simulink model "Compliance"  (R2020b)
settings: Solver=VariableStepAuto  StartTime=0.0  StopTime=3  RelTol=1e-3
values from neighbouring files (symbols this model uses):
  K = 10*diag([1 1 30 1 1 1])    [parameters.m]
  KD = diag([  150   180   160    19     0   8])    [parameters.m]
  KP = diag([1700  3000  1600  100  1  4])    [parameters.m]
libraries: vrlib x1
settings Model: Creator=Edoardo  LastModifiedBy=Edoardo

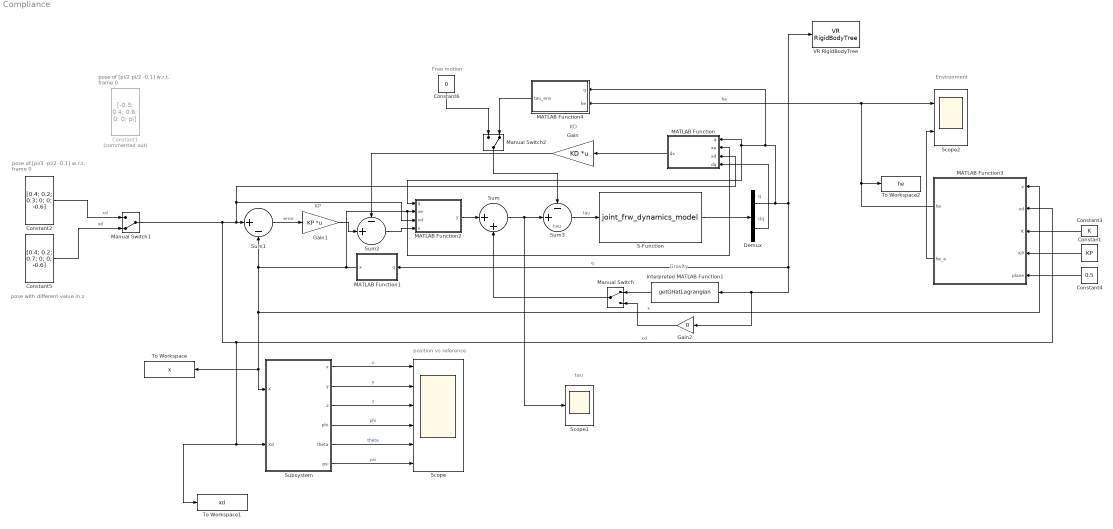
== system Compliance ==
  note: Free motion
  note: Environment
  note: tau
  note: Gravity
  note: tau
  note: KP
  note: KD
  note: dq
  note: q
  note: position vs reference
  note: pose of [pi/2 pi/2 -0.1]
      | w.r.t. frame 0
  note: pose of [pi/3 -pi/2 -0.1]
      | w.r.t. frame 0
  note: pose with different value in z
  Constant : Constant  Value=KP
  Constant1 : Constant  Commented=on  Value=[-0.3; 0.4; 0.6; 0; 0; pi]  VectorParams1D=off
  Constant2 : Constant  Value=[0.4; 0.2; 0.3; 0; 0; -0.6]  VectorParams1D=off
  Constant3 : Constant  Value=K
  Constant4 : Constant  Value=0.5
  Constant5 : Constant  Value=[0.4; 0.2; 0.7; 0; 0; -0.6]  VectorParams1D=off
  Constant6 : Constant  Value=0
  Demux : Demux  Outputs=2
  Gain : Gain  Gain=KD  Multiplication=Matrix(K*u) (u vector)
  Gain1 : Gain  Gain=KP  Multiplication=Matrix(K*u) (u vector)
  Gain2 : Gain  Gain=0
  Interpreted MATLAB Function1 : MATLABFcn  MATLABFcn=getGHatLagrangian
  MATLAB Function : MATLAB Function  TreatAsAtomicUnit=on
  MATLAB Function1 : MATLAB Function  TreatAsAtomicUnit=on
  MATLAB Function2 : MATLAB Function  TreatAsAtomicUnit=on
  MATLAB Function3 : MATLAB Function  TreatAsAtomicUnit=on
  MATLAB Function4 : MATLAB Function  TreatAsAtomicUnit=on
  Manual Switch : ManualSwitch
  Manual Switch1 : ManualSwitch  CurrentSetting=0
  Manual Switch2 : ManualSwitch  CurrentSetting=0
  S-Function : S-Function  FunctionName=joint_frw_dynamics_model  Parameters=myRobot  SFunctionDeploymentMode=off  EnableBusSupport=off
  Scope : Scope  NumInputPorts=6
  Scope1 : Scope
  Scope2 : Scope  NumInputPorts=2
  Subsystem : Subsystem
  Sum : Sum  Inputs=|++
  Sum1 : Sum  Inputs=|+-
  Sum2 : Sum  Inputs=-+|
  Sum3 : Sum  Inputs=-+|
  To Workspace : ToWorkspace  VariableName=x  SaveFormat=Timeseries  SampleTime=-1
  To Workspace1 : ToWorkspace  VariableName=xd  SaveFormat=Timeseries  SampleTime=-1
  To Workspace2 : ToWorkspace  VariableName=he  SaveFormat=Timeseries  SampleTime=-1
  VR RigidBodyTree : vrlib/VR RigidBodyTree  RBT=robot  useRBT=on  Ts=-1  ForceViewerOpen=on
      settings: SourceProductBaseCode=SL
  wires:
  S-Function/1 -> Demux/1
  Sum/1 -> Sum3/2, Scope1/1
  Gain/1 -> Sum2/1
  Sum1/1 -> Gain1/1  "error"
  Demux/1 -> MATLAB Function/1(q), MATLAB Function2/1(q), MATLAB Function4/1(q), VR RigidBodyTree/1, Gain2/1, Interpreted MATLAB Function1/1, MATLAB Function1/1(q)  "q"
  Gain1/1 -> Sum2/2
  Manual Switch1/1 -> MATLAB Function2/3(xd), MATLAB Function/3(xd), Sum1/1, MATLAB Function3/2(xd), To Workspace1/1, Subsystem/2(Xd)  "xd"
  Gain2/1 -> Manual Switch/2
  Interpreted MATLAB Function1/1 -> Manual Switch/1
  Demux/2 -> MATLAB Function/4(dq)
  MATLAB Function/1(dx) -> Gain/1
  MATLAB Function1/1(x) -> MATLAB Function/2(xe), MATLAB Function2/2(xe), Subsystem/1(X), To Workspace/1, MATLAB Function3/1(x), Sum1/2  "x"
  Sum2/1 -> MATLAB Function2/4(x)
  Subsystem/1(x) -> Scope/1  "x"
  Subsystem/2(y) -> Scope/2  "y"
  Subsystem/3(z) -> Scope/3  "z"
  Subsystem/4(phi) -> Scope/4  "phi"
  Subsystem/5(theta) -> Scope/5  "theta"
  Subsystem/6(psi) -> Scope/6  "psi"
  Manual Switch/1 -> Sum/2
  MATLAB Function3/1(he) -> MATLAB Function4/2(he), Scope2/1, To Workspace2/1  "he"
  Constant/1 -> MATLAB Function3/4(KP)
  Constant4/1 -> MATLAB Function3/5(plane)
  Constant3/1 -> MATLAB Function3/3(K)
  Sum3/1 -> S-Function/1  "tau"
  MATLAB Function2/1(y) -> Sum/1
  Constant2/1 -> Manual Switch1/1  "xd"
  Constant5/1 -> Manual Switch1/2  "xd"
  MATLAB Function3/2(he_e) -> Scope2/2
  Manual Switch2/1 -> Sum3/1
  MATLAB Function4/1(tau_env) -> Manual Switch2/2
  Constant6/1 -> Manual Switch2/1

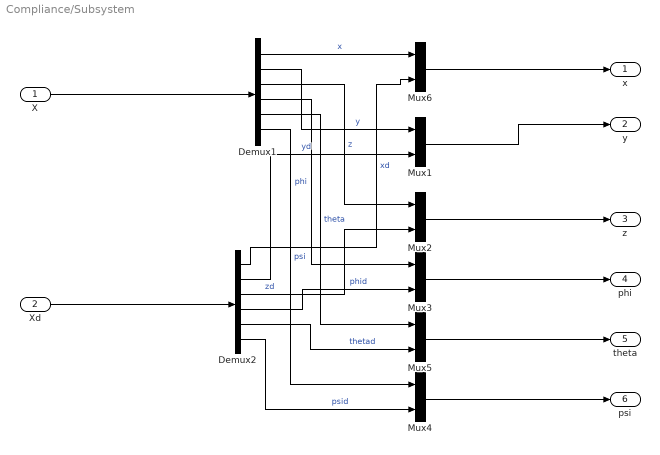
== system Compliance/Subsystem ==
  X : Inport
  Xd : Inport  Port=2
  Demux1 : Demux  Outputs=6
  Demux2 : Demux  Outputs=6
  Mux{1..6} (6 alike) : Mux  Inputs=2
  x : Outport
  y : Outport  Port=2
  z : Outport  Port=3
  phi : Outport  Port=4
  theta : Outport  Port=5
  psi : Outport  Port=6
  wires:
  Demux1/3 -> Mux2/1  "z"
  Demux1/4 -> Mux3/1  "phi"
  Demux2/3 -> Mux2/2  "zd"
  Mux2/1 -> z/1
  Demux2/1 -> Mux6/2  "xd"
  Demux1/5 -> Mux5/1  "theta"
  Mux1/1 -> y/1
  Demux1/6 -> Mux4/1  "psi"
  Demux1/1 -> Mux6/1  "x"
  Demux2/5 -> Mux5/2  "thetad"
  Demux2/6 -> Mux4/2  "psid"
  Demux1/2 -> Mux1/1  "y"
  Demux2/4 -> Mux3/2  "phid"
  Demux2/2 -> Mux1/2  "yd"
  Xd/1 -> Demux2/1
  X/1 -> Demux1/1
  Mux3/1 -> phi/1
  Mux5/1 -> theta/1
  Mux4/1 -> psi/1
  Mux6/1 -> x/1

== matlab function Compliance/MATLAB Function1 ==
  data: q input size=3; x output size=6
function x = K(q)

K = getDirectKinematics(q);

pos = K(1:3, 4);
rotm = K(1:3,1:3); 
ori = rotm2eul(rotm, 'ZYZ')';

x = [pos; ori];

== matlab function Compliance/MATLAB Function ==
  data: q input size=3; xe input; xd input; dx output size=6; dq input size=3
function dx = JAd(q,xe, xd, dq)

Re = eul2rotm(xe(4:6)', 'ZYZ');
Rd = eul2rotm(xd(4:6)', 'ZYZ');
Te = zeros(4,4);
Te(1:3, 1:3) = Re;
Te(1:3, 4) = xe(1:3);
Te(4,4) = 1;

Td = zeros(4,4);
Td(1:3, 1:3) = Rd;
Td(1:3, 4) = xd(1:3);
Td(4,4) = 1;
   
Tde = inv(Td)*Te;
phide = rotm2eul(Tde(1:3, 1:3), 'ZYZ');

% Compute the rotational matrix of the desired fame xd
Rde = eul2rotm(xd(4:6)', 'ZYZ');

% Compute the analytical jacobian respect to the desired frame 
Jad = pinv(getTransformAnalytical(phide))*[Rde', zeros(3,3); zeros(3,3), Rde']*getJacobian(q);

dx = Jad*dq;

== matlab function Compliance/MATLAB Function2 ==
  data: q input size=3; xe input; xd input; y output size=3; x input
function y = JAdT(q,xe, xd, x)

Re = eul2rotm(xe(4:6)', 'ZYZ');
Rd = eul2rotm(xd(4:6)', 'ZYZ');

Te = zeros(4,4);
Te(1:3, 1:3) = Re;
Te(1:3, 4) = xe(1:3);
Te(4,4) = 1;

Td = zeros(4,4);
Td(1:3, 1:3) = Rd;
Td(1:3, 4) = xd(1:3);
Td(4,4) = 1;
   
Tde = inv(Td)*Te;
phide  = rotm2eul(Tde(1:3, 1:3), 'ZYZ');


% Compute the rotational matrix of the desired fame xd
Rd = eul2rotm(xd(4:6)', 'ZYZ');

% Compute the analytical jacobian respect to the desired frame 
Jad = pinv(getTransformAnalytical(phide))*[Rd', zeros(3,3); zeros(3,3), Rd']*getJacobian(q);

y = Jad'*x;

== matlab function Compliance/MATLAB Function3 ==
  data: x input; he output; xd input; K input; KP input; plane input; he_e output
function [he, he_e]   = environment(x, xd, K, KP, plane)

% the robot is touching the environment!
if x(3) >= plane 
    
    % set up the rest position frame
    xr = zeros(6,1);
    xr(3) = plane;
    
    % compute the forces
    %dx_rd = xd - xr;
    dx_rd = zeros(6,1);
    dx_rd(3) = xd(3) - xr(3);
    
    
    xe = zeros(6,1);
    xe(3) = x(3);

    he = K * (xe - xr);
    
    he_e_total =  K/(eye(6) + K / KP) * dx_rd;
    he_e = he_e_total(2); 
    dx_ed = KP \ he;
   
% free motion
else
    
    he = zeros(6,1);
    he_e = 0;
    dx_ed = zeros(6,1);
end

== matlab function Compliance/MATLAB Function4 ==
  data: q input; he input; tau_env output
function tau_env = JT(q, he)

tau_env = getJacobian(q)'*he;
